simulink model "TRK_1a"  (R2026a)
settings: Solver=ode4  StopTime=1700  FixedStep=0.005
InitFcn:
  | TRK
values from neighbouring files (symbols this model uses):
  K_scheduled = zeros(length(V_op), 2)    [CAL3.m]    (also in CUB.m; DLC2.m; MUS.m; OHZ.m)
  V_op = 5:5:85    [CAL3.m]    (also in CUB.m; DLC2.m; MUS.m; OHZ.m)
  V_track = vx_scaled    [TRK.m]
  X_track = [linspace(0, runway_length, 200)'; runway_length + R_track * cos(theta_circ(2:end))]    [CAL3.m]    (also in CUB.m = [0; 5000]; DLC2.m = 0:0.1:total_track_length; MUS.m = [0; 2000]; OHZ.m = [0; 2000])
  Y_track = [zeros(200, 1); R_track + R_track * sin(theta_circ(2:end))]    [CAL3.m]    (also in CUB.m = [0; 0]; DLC2.m = zeros(size(X_track)); MUS.m = [0; 0]; OHZ.m = [0; 0])
undefined symbols (not defined in the file or in its folder): sim_params
libraries: sl_discontinuities x1, slpidlib x1, simulink x1
(part 2 of 2)

== matlab function TRK_1a/Scopes1/MATLAB Function ==
  settings: updateMethod=DISCRETE
  data: X_curr input; Y_curr input; psi_curr input; vx_curr input; delta_curr input; t_curr input; X_track parameter; Y_track parameter
function live_track_plotter(X_curr, Y_curr, psi_curr, vx_curr, delta_curr, t_curr, X_track, Y_track)
    coder.extrinsic('figure', 'plot', 'hold', 'axis', 'title', 'xlabel', 'ylabel', 'set', 'drawnow', 'legend', 'grid', 'patch', 'text');
    
    persistent hFig hCar hText counter 
    persistent hTimers lap_count lap_start_time lap_trigger_ready past_laps
    persistent trail_X trail_Y trail_idx hTrailLine 
    
    % --- DOTTED LINE FIX ---
    % Downsample the visual track by taking every 50th point.
    % This stops the dashes from overlapping so the dotted line appears correctly.
    X_ref = X_track(1:50:end);
    Y_ref = Y_track(1:50:end);
    
    origin_X = X_track(1);
    origin_Y = Y_track(1);
    
    if isempty(counter)
        counter = 0;
        lap_count = 1;
        lap_start_time = 0;
        lap_trigger_ready = false;
        
        past_laps = zeros(1, 10);
        hTimers = zeros(1, 10);
        
        % Preallocate trail with NaNs (Fastest method for MATLAB renderer)
        trail_X = nan(1, 200000); 
        trail_Y = nan(1, 200000);
        trail_idx = 1;
        
        hFig = figure('Name', 'Live Telemetry: Monza', 'Color', 'w', 'Position', [100, 100, 800, 600]);
        
        % Plot the downsampled reference line
        hRef = plot(X_ref, Y_ref, '--', 'Color', [0.4 0.4 0.4], 'LineWidth', 1.5); hold on;
        hStart = plot(origin_X, origin_Y, 'ko', 'MarkerSize', 10, 'MarkerFaceColor', 'g', 'LineWidth', 1.5);
        
        text(origin_X - 50, origin_Y + 70, 'Start / Finish', 'FontSize', 10, 'FontWeight', 'bold', 'Color', 'k', 'BackgroundColor', [1 1 1 0.7]);
        
        % Initialize the single Trail Line and Car Patch
        hTrailLine = double(plot(trail_X, trail_Y, 'b-', 'LineWidth', 1.5));
        hCar = double(patch(0, 0, [0.8 0 0], 'EdgeColor', 'k', 'LineWidth', 1));
        set(hCar, 'FaceAlpha', 0.8); 
        
        hText = text(0, 0, ' Init...', 'FontSize', 10, 'FontWeight', 'bold', 'BackgroundColor', [1 1 1 0.8], 'EdgeColor', 'k', 'Margin', 2);
        
        box_props = {'Units', 'normalized', 'HorizontalAlignment', 'right', 'FontSize', 11, 'FontWeight', 'bold', 'BackgroundColor', [1 1 1 0.9], 'EdgeColor', 'k', 'Margin', 3, 'Visible', 'off'};
        
        for i = 1:10
            y_pos = 0.95 - ((i - 1) * 0.045);
            hTimers(i) = double(text(0.95, y_pos, '', box_props{:}));
        end
        
        axis equal; grid on;
        title('Live Vehicle Tracking with Telemetry');
        xlabel('X Position (meters)'); ylabel('Y Position (meters)');
        
        legend([hRef, hStart, hTrailLine, hCar], {'Reference Track', 'Start/Finish', 'Driven Path', 'EV Position'}, 'Location', 'best', 'AutoUpdate', 'off');
    end
    
    counter = counter + 1;
    
    % --- LAP TIMING LOGIC ---
    dist_to_origin = sqrt((X_curr - origin_X)^2 + (Y_curr - origin_Y)^2);
    
    if dist_to_origin > 50
        lap_trigger_ready = true;
    end
    
    if lap_trigger_ready && dist_to_origin < 15
        if lap_count <= 10
            past_laps(lap_count) = t_curr - lap_start_time;
        end
        
        lap_count = lap_count + 1;
        lap_start_time = t_curr;
        lap_trigger_ready = false; 
    end
    
    % --- SPEED FIX: UPDATE UI AT 20Hz INSTEAD OF 100Hz ---
    if mod(counter, 50) == 0
        
        % UPDATE TRAIL
        if trail_idx <= 200000
            trail_X(trail_idx) = X_curr;
            trail_Y(trail_idx) = Y_curr;
            trail_idx = trail_idx + 1;
        end
        
        % Push the NaN array directly (highly optimized in MATLAB backend)
        set(hTrailLine, 'XData', trail_X, 'YData', trail_Y);
        
        % --- SCALING ---
        L_vis = 4.5; 
        W_vis = 1.9; 
        
        base_X = [L_vis/2,  L_vis*0.3,   0,       -L_vis*0.35, -L_vis/2,  -L_vis/2,   -L_vis*0.35,  0,        L_vis*0.3,   L_vis/2];
        base_Y = [0,        W_vis*0.45, W_vis/2,  W_vis/2,     W_vis*0.3, -W_vis*0.3, -W_vis/2,    -W_vis/2, -W_vis*0.45, 0];
        
        R = [cos(psi_curr), -sin(psi_curr); 
             sin(psi_curr),  cos(psi_curr)];
             
        rotated_coords = R * [base_X; base_Y];
        final_X = rotated_coords(1, :) + X_curr;
        final_Y = rotated_coords(2, :) + Y_curr;
        
        set(hCar, 'XData', final_X, 'YData', final_Y);
        
        % Update Floating Telemetry Text
        speed_kmh = vx_curr * 3.6;
        steer_deg = delta_curr * (180 / pi);
        
        telemetry_str = sprintf(' Spd: %.1f km/h\n Steer. Ang.: %.1f deg', speed_kmh, steer_deg);
        set(hText, 'Position', [X_curr + 15, Y_curr + 15], 'String', telemetry_str);
        
        % --- UPDATE LAP TIMERS ---
        current_live_time = t_curr - lap_start_time;
        
        for i = 1:10
            if i < lap_count
                set(hTimers(i), 'String', sprintf(' Lap %d: %d:%06.3f ', int32(i), int32(floor(past_laps(i)/60)), mod(past_laps(i), 60)), 'Visible', 'on');
            elseif i == lap_count
                set(hTimers(i), 'String', sprintf(' Lap %d: %d:%06.3f (Live) ', int32(i), int32(floor(current_live_time/60)), mod(current_live_time, 60)), 'Visible', 'on', 'Color', [0 0 0.8]);
            end
        end
        
        drawnow limitrate; 
    end
end

== matlab function TRK_1a/Vehicle Control Unit (VCU)1/MATLAB Function ==
  settings: updateMethod=DISCRETE
  data: delta_curr input; pedal input; T_rr_motor_raw output size=1; vx_curr input; vy_curr input; r_curr input; kappa_ref input; Fz_f_total input; Fz_r_total input; Fz_rl input; Fz_rr input; SOC input; T_batt input; T_motor input; V_op parameter; K_scheduled parameter; T_rl_motor_raw output size=1; T_rr_fric output size=1; w_vec input; T_rl_fric output size=1; T_f_fric output size=1; Mz_cmd output size=1; r_ref output size=1
function [T_rr_motor_raw, T_rl_motor_raw, T_rr_fric, T_rl_fric, T_f_fric, Mz_cmd, r_ref] = vcu_allocator(delta_curr, pedal, vx_curr, vy_curr, r_curr, kappa_ref, Fz_f_total, Fz_r_total, Fz_rl, Fz_rr, SOC, T_batt, T_motor, V_op, K_scheduled, w_vec)

% --- INITIALIZATION (Satisfying the Coder) ---
T_rr_motor_raw = 0.0;
T_rl_motor_raw = 0.0;
T_rr_fric = 0.0;
T_rl_fric = 0.0;
T_f_fric = 0.0;
Mz_cmd = 0.0;
r_ref = 0.0;

Rw = 0.34; tw = 1.65; G = 10; mu_max = 1.2;

% --- Limits & Derating ---
P_motor_base = 250000; 
T_motor_max = 400;     
T_fric_max_per_wheel = 3500;

T_batt_cal = [-10, 0, 15, 45, 55, 60]; 
P_derate_batt_cal = [0, 0.5, 1.0, 1.0, 0.2, 0];
T_motor_cal = [30, 90, 110, 130, 150]; 
P_derate_motor_cal = [1.0, 1.0, 1.0, 1.0, 0.5];
SOC_vec = [0, 0.05, 0.15, 0.85, 0.95, 1.0]; 
P_derate_SOC_dis = [0, 0.1, 1.0, 1.0, 1.0, 1.0]; 
P_derate_SOC_chg = [1.0, 1.0, 1.0, 1.0, 0.1, 0];
    
derate_T_batt = interp1(T_batt_cal, P_derate_batt_cal, T_batt(1), 'linear', 0);
derate_T_mot = interp1(T_motor_cal, P_derate_motor_cal, T_motor(1), 'linear', 0);
derate_T_total = min(derate_T_batt, derate_T_mot);
derate_S_dis = interp1(SOC_vec, P_derate_SOC_dis, SOC(1), 'linear', 0);
derate_S_chg = interp1(SOC_vec, P_derate_SOC_chg, SOC(1), 'linear', 0);

P_avail_dis = P_motor_base * min(derate_T_total, derate_S_dis);
P_avail_chg = P_motor_base * min(derate_T_total, derate_S_chg);

vx_lqr = max(vx_curr(1), 5.0);

% --- Torque Vectoring Blending ---
vx_kmh = vx_curr(1) * 3.6;
tv_blend_lower = 45.0;
tv_blend_upper = 50.0;
if vx_kmh >= tv_blend_upper
    tv_blend = 1.0;
elseif vx_kmh <= tv_blend_lower
    tv_blend = 0.0;
else
    tv_blend = (vx_kmh - tv_blend_lower) / (tv_blend_upper - tv_blend_lower);
end

% --- LQR Yaw Moment Calculation ---
K_dyn_1 = interp1(V_op, K_scheduled(:,1), vx_lqr, 'linear', 'extrap');
K_dyn_2 = interp1(V_op, K_scheduled(:,2), vx_lqr, 'linear', 'extrap');

L = 2.6;            
K_us = 0.0015;      
g = 9.81;

r_ref_raw = (vx_lqr * delta_curr(1)) / (L * (1 + K_us * vx_lqr^2));
r_max_phys = (mu_max * g * 0.95) / vx_lqr;

% Assigning to output variable
r_ref = max(-r_max_phys, min(r_max_phys, r_ref_raw));

TV_Bite_Factor = 1;
vy_factor = 1;
Mz_req = tv_blend * -(vy_factor * K_dyn_1(1) * vy_curr(1) + TV_Bite_Factor * K_dyn_2(1) * (r_curr(1) - r_ref));

% Assigning to output variable directly
Mz_cmd = max(-2500, min(2500, Mz_req(1)));
T_delta_wheel_raw = max(-1500, min(1500, (Mz_cmd * Rw) / tw));

% --- DYNAMIC MOTOR POWER LIMITS ---
w_motor_rl = max(abs(w_vec(3) * G), 0.1); 
w_motor_rr = max(abs(w_vec(4) * G), 0.1);

T_limit_rl_dis = P_avail_dis / ((1)*w_motor_rl);
T_limit_rr_dis = P_avail_dis / ((1)*w_motor_rr);
T_limit_rl_chg = P_avail_chg / ((1)*w_motor_rl);
T_limit_rr_chg = P_avail_chg / ((1)*w_motor_rr);

T_motor_lim_rl_dis = min(T_motor_max, T_limit_rl_dis);
T_motor_lim_rr_dis = min(T_motor_max, T_limit_rr_dis);
T_motor_lim_rl_chg = max(-T_motor_max, -T_limit_rl_chg);
T_motor_lim_rr_chg = max(-T_motor_max, -T_limit_rr_chg);

T_grip_lim_rl_wheel = mu_max * Fz_rl(1) * Rw * 0.90;
T_grip_lim_rr_wheel = mu_max * Fz_rr(1) * Rw * 0.90;

T_max_rl_motor = min(T_motor_lim_rl_dis, T_grip_lim_rl_wheel / G);
T_max_rr_motor = min(T_motor_lim_rr_dis, T_grip_lim_rr_wheel / G);
T_min_rl_motor = max(T_motor_lim_rl_chg, -T_grip_lim_rl_wheel / G);
T_min_rr_motor = max(T_motor_lim_rr_chg, -T_grip_lim_rr_wheel / G);

weight_rl = Fz_rl(1) / max(1, (Fz_rl(1) + Fz_rr(1)));
weight_rr = Fz_rr(1) / max(1, (Fz_rl(1) + Fz_rr(1)));

% --- DRIVE / BRAKE MODE ROUTING ---
if pedal(1) >= 0
    T_req_total_motor = pedal(1) * (T_max_rl_motor + T_max_rr_motor);
    T_rr_base_motor = T_req_total_motor * weight_rr;
    T_rl_base_motor = T_req_total_motor * weight_rl;
    
    T_rr_motor_raw = max(T_min_rr_motor, min(T_max_rr_motor, T_rr_base_motor + (T_delta_wheel_raw/G)));
    T_rl_motor_raw = max(T_min_rl_motor, min(T_max_rl_motor, T_rl_base_motor - (T_delta_wheel_raw/G)));
    
    v_hub_rl = max(vx_curr(1) - (tw/2)*r_curr(1), 1.0);
    v_hub_rr = max(vx_curr(1) + (tw/2)*r_curr(1), 1.0);
    
    kappa_rl = (w_vec(3)*Rw - v_hub_rl) / v_hub_rl;
    kappa_rr = (w_vec(4)*Rw - v_hub_rr) / v_hub_rr;
    
    slip_target = 0.10;
    Kp_tcs = 1000;
    worst_kappa_rear = max(kappa_rl, kappa_rr);
    
    if worst_kappa_rear > slip_target
        T_tcs_penalty = Kp_tcs * (worst_kappa_rear - slip_target);
        T_rl_motor_raw = max(0, T_rl_motor_raw - T_tcs_penalty);
        T_rr_motor_raw = max(0, T_rr_motor_raw - T_tcs_penalty);
    end
    
    T_rr_fric = 0.0; 
    T_rl_fric = 0.0; 
    T_f_fric = 0.0;

else
    bias_f = 0.70;
    total_grip_cap_wheel = mu_max * (Fz_f_total(1) + Fz_r_total(1)) * Rw * 0.90;
    
    T_req_total_wheel = pedal(1) * total_grip_cap_wheel;
    T_req_front_wheel = T_req_total_wheel * bias_f;
    T_req_rear_wheel  = T_req_total_wheel * (1 - bias_f);
    
    T_f_fric = max(-mu_max * Fz_f_total(1) * Rw * 0.90, T_req_front_wheel);
    
    T_base_rr = max(-(T_grip_lim_rr_wheel - abs(T_delta_wheel_raw)), T_req_rear_wheel * weight_rr);
    T_base_rl = max(-(T_grip_lim_rl_wheel - abs(T_delta_wheel_raw)), T_req_rear_wheel * weight_rl);
    
    T_rr_ideal_wheel = T_base_rr + T_delta_wheel_raw;
    T_rl_ideal_wheel = T_base_rl - T_delta_wheel_raw;
    
    v_hub_fl = max(vx_curr(1) - (tw/2)*r_curr(1), 1.0);
    v_hub_fr = max(vx_curr(1) + (tw/2)*r_curr(1), 1.0);
    v_hub_rl = max(vx_curr(1) - (tw/2)*r_curr(1), 1.0);
    v_hub_rr = max(vx_curr(1) + (tw/2)*r_curr(1), 1.0);
    
    kappa_fl = (w_vec(1)*Rw - v_hub_fl) / v_hub_fl;
    kappa_fr = (w_vec(2)*Rw - v_hub_fr) / v_hub_fr;
    kappa_rl = (w_vec(3)*Rw - v_hub_rl) / v_hub_rl;
    kappa_rr = (w_vec(4)*Rw - v_hub_rr) / v_hub_rr;
    
    slip_limit_abs = -0.10;
    Kp_abs = 5000;
    
    worst_kappa_f = min(kappa_fl, kappa_fr);
    if worst_kappa_f < slip_limit_abs
        T_f_fric = min(0.0, T_f_fric - Kp_abs * (worst_kappa_f - slip_limit_abs));
    end
    
    if kappa_rl < slip_limit_abs
        T_rl_ideal_wheel = min(0.0, T_rl_ideal_wheel - Kp_abs * (kappa_rl - slip_limit_abs));
    end
    if kappa_rr < slip_limit_abs
        T_rr_ideal_wheel = min(0.0, T_rr_ideal_wheel - Kp_abs * (kappa_rr - slip_limit_abs));
    end
    
    T_rr_motor_raw = max(T_min_rr_motor, min(T_max_rr_motor, T_rr_ideal_wheel / G));
    T_rl_motor_raw = max(T_min_rl_motor, min(T_max_rl_motor, T_rl_ideal_wheel / G));
    
    T_rr_fric = max(-T_fric_max_per_wheel, min(0.0, T_rr_ideal_wheel - (T_rr_motor_raw * G)));
    T_rl_fric = max(-T_fric_max_per_wheel, min(0.0, T_rl_ideal_wheel - (T_rl_motor_raw * G)));
    
    if vx_curr(1) < 2.0
        T_f_fric = 0.0; 
        T_rr_fric = 0.0; 
        T_rl_fric = 0.0;
        T_rr_motor_raw = 0.0; 
        T_rl_motor_raw = 0.0;
    end
end

% =========================================================================
% FINAL ENFORCEMENT (Satisfying Copilot)
% =========================================================================
T_rr_motor_raw = double(T_rr_motor_raw(1));
T_rl_motor_raw = double(T_rl_motor_raw(1));
T_rr_fric      = double(T_rr_fric(1));
T_rl_fric      = double(T_rl_fric(1));
T_f_fric       = double(T_f_fric(1));
Mz_cmd         = double(Mz_cmd(1));
r_ref          = double(r_ref(1));

end
